simulink library "sixDoFDynamicsCoupled2"  (R2020a)
settings: Solver=VariableStepAuto  StartTime=0.0  StopTime=10.0  RelTol=1e-3
undefined symbols (not defined in the file): vcl
libraries: vrlib x8, eulAng2RotMat_ul x1, eulDot x1
settings Model: Creator=jldanie5  LastModifiedBy=John Jr
settings DataIOCC: ReturnWorkspaceOutputs=off
settings DebuggingCC: ArithmeticOperatorsInVariantConditions=warning
settings SFSimCC: CustomCodeUndefinedFunction=UseInterfaceOnly

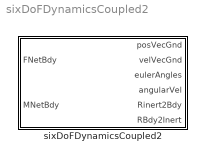
== system sixDoFDynamicsCoupled2 ==
  sixDoFDynamicsCoupled2 : Subsystem  VariantControl=(default)  mask{MMat=vcl.M6x6_B.Value, MaMat=vcl.Ma6x6_LE.Value, rCM_B=vcl.rCM_B.Value, rB_LE=vcl.rB_LE.Value, initPos=vcl.initPosVecGnd.Value, initVel=vcl.initVelVecBdy.Value, initEulAngs=vcl.initEulAng.Value, initAngVel=vcl.initAngVelVec.Value}
      mask prompts: MMat "6x6 Mass Matrix"; MaMat "6x6 Added Mass Matrix"; rCM_B "Center of mass position vec in body frame"; rB_LE "Body frame origin position vec relative to Leading Edge"; initPos "Initial position"; initVel "Initial velocity"; initEulAngs "Initial Euler Angles"; initAngVel "Initial Angular Velocity Vec"
      mask init:
      | S = @(v) [0 -v(3) v(2);v(3) 0 -v(1);-v(2) v(1) 0];
      | MaAdj = [eye(3) zeros(3);-S(rB_LE) eye(3)]*MaMat;
      | MTot = MMat + MaAdj;
      | MTotInv = inv(MTot);
      | 
      | m = MMat(1,1);
      | J = MMat(4:6,4:6);%About Body Frame
      mask DialogControl Container6 Prompt: Mass Matrices
      mask DialogControl Container4 Prompt: Point Locations
      mask DialogControl Container3 Prompt: Initial Conditions

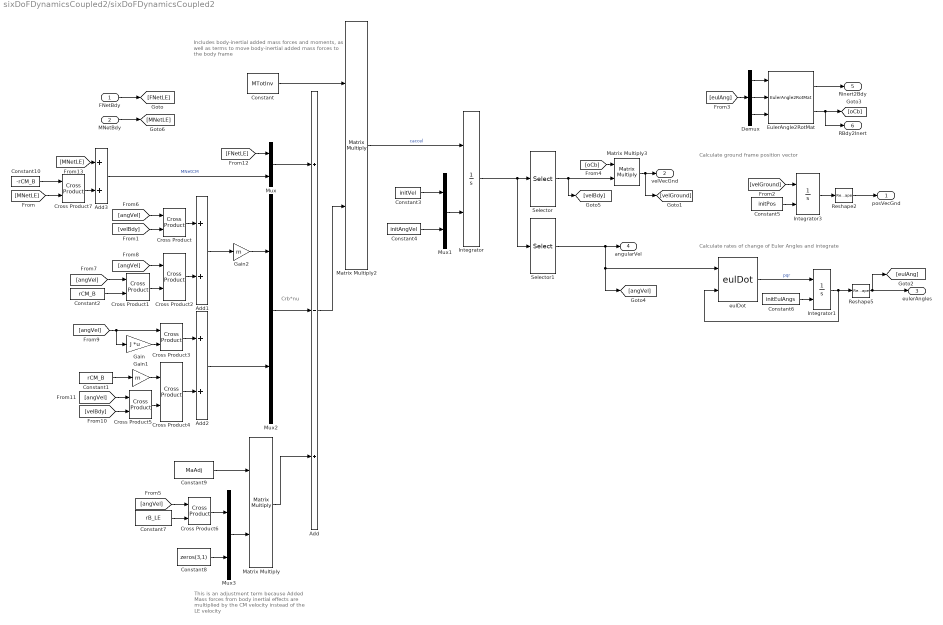
== system sixDoFDynamicsCoupled2/sixDoFDynamicsCoupled2 ==
  note: Crb*nu
  note: This is an adjustment term because Added
      | Mass forces from body inertial effects are
      | multiplied by the CM velocity instead
      | of the LE velocity
  note: Includes body-inertial added mass forces and moments,
      | as well as terms to move body-inertial added mass
      | forces to the body frame
  note: Calculate ground frame position vector
  note: Calculate rates of change of Euler Angles and integrate
  FNetBdy : Inport
  MNetBdy : Inport  Port=2
  Add : Sum  Inputs=+-+
  Add1 : Sum
  Add2 : Sum
  Add3 : Sum
  Constant : Constant  Value=MTotInv  VectorParams1D=off
  Constant1 : Constant  Value=rCM_B
  Constant10 : Constant  Value=-rCM_B  VectorParams1D=off
  Constant2 : Constant  Value=rCM_B
  Constant3 : Constant  Value=initVel
  Constant4 : Constant  Value=initAngVel
  Constant5 : Constant  Value=initPos
  Constant6 : Constant  Value=initEulAngs
  Constant7 : Constant  Value=rB_LE
  Constant8 : Constant  Value=zeros(3,1)
  Constant9 : Constant  Value=MaAdj
  Cross Product{,1..7} (8 alike) : vrlib/Utilities/Cross Product
  Demux : Demux  Outputs=3
  EulerAngle2RotMat : eulAng2RotMat_ul/EulerAngle2RotMat  SystemSampleTime=-1  Latency=0  AutoFrameSizeCalculation=off
  Gain : Gain  Gain=J  Multiplication=Matrix(K*u)
  Gain1 : Gain  Gain=m
  Gain2 : Gain  Gain=m
  Integrator : Integrator  InitialConditionSource=external
  Integrator1 : Integrator  InitialConditionSource=external  InitialCondition=initEulAngs
  Integrator3 : Integrator  InitialConditionSource=external  InitialCondition=initPos
  Matrix Multiply : Product  Multiplication=Matrix(*)
  Matrix Multiply2 : Product  Multiplication=Matrix(*)
  Matrix Multiply3 : Product  Multiplication=Matrix(*)
  Mux{,1..3} (4 alike) : Mux  Inputs=2
  Reshape2 : Reshape  OutputDimensionality=Column vector (2-D)
  Reshape5 : Reshape  OutputDimensionality=Column vector (2-D)
  Selector : Selector  InputPortWidth=6  IndexOptions=Index vector (dialog)  Indices=[1 2 3]  OutputSizes=1
  Selector1 : Selector  InputPortWidth=6  IndexOptions=Index vector (dialog)  Indices=[4 5 6]  OutputSizes=1
  eulDot : eulDot/eulDot  SystemSampleTime=-1  Latency=0  AutoFrameSizeCalculation=off
  posVecGnd : Outport  VectorParamsAs1DForOutWhenUnconnected=off
  velVecGnd : Outport  Port=2  VectorParamsAs1DForOutWhenUnconnected=off
  eulerAngles : Outport  Port=3  VectorParamsAs1DForOutWhenUnconnected=off
  angularVel : Outport  Port=4  VectorParamsAs1DForOutWhenUnconnected=off
  Rinert2Bdy : Outport  Port=5  VectorParamsAs1DForOutWhenUnconnected=off
  RBdy2Inert : Outport  Port=6  VectorParamsAs1DForOutWhenUnconnected=off
  wires:
  Mux/1 -> Add/1
  Constant/1 -> Matrix Multiply2/1
  Matrix Multiply2/1 -> Integrator/1  "caccel"
  Integrator/1 -> Selector1/1, Selector/1
  Constant4/1 -> Mux1/2
  Mux1/1 -> Integrator/2
  Integrator3/1 -> Reshape2/1
  Demux/3 -> EulerAngle2RotMat/3
  Demux/1 -> EulerAngle2RotMat/1
  EulerAngle2RotMat/2 -> RBdy2Inert/1, [oCb]
  Reshape2/1 -> posVecGnd/1
  Demux/2 -> EulerAngle2RotMat/2
  Constant5/1 -> Integrator3/2
  [eulAng] -> Demux/1
  eulDot/1 -> Integrator1/1  "pqr"
  Integrator1/1 -> Reshape5/1, eulDot/2
  Constant6/1 -> Integrator1/2
  Reshape5/1 -> eulerAngles/1, [eulAng]
  Selector1/1 -> [angVel], eulDot/1, angularVel/1
  [velGround] -> Integrator3/1
  EulerAngle2RotMat/1 -> Rinert2Bdy/1
  Constant3/1 -> Mux1/1
  Selector/1 -> [velBdy], Matrix Multiply3/2
  [oCb] -> Matrix Multiply3/1
  Matrix Multiply3/1 -> [velGround], velVecGnd/1
  Mux2/1 -> Add/2
  [velBdy] -> Cross Product/2
  [angVel] -> Cross Product/1
  Cross Product/1 -> Add1/1
  Cross Product1/1 -> Cross Product2/2
  Constant2/1 -> Cross Product1/2
  [angVel] -> Cross Product1/1
  [angVel] -> Cross Product2/1
  Cross Product2/1 -> Add1/2
  [angVel] -> Cross Product3/1, Gain/1
  Gain/1 -> Cross Product3/2
  Constant1/1 -> Gain1/1
  Gain1/1 -> Cross Product4/1
  [velBdy] -> Cross Product5/2
  [angVel] -> Cross Product5/1
  Cross Product5/1 -> Cross Product4/2
  Cross Product3/1 -> Add2/1
  Cross Product4/1 -> Add2/2
  Add1/1 -> Gain2/1
  Add2/1 -> Mux2/2
  Add/1 -> Matrix Multiply2/2
  Gain2/1 -> Mux2/1
  Matrix Multiply/1 -> Add/3
  [angVel] -> Cross Product6/1
  Constant7/1 -> Cross Product6/2
  Cross Product6/1 -> Mux3/1
  Constant8/1 -> Mux3/2
  Mux3/1 -> Matrix Multiply/2
  Constant9/1 -> Matrix Multiply/1
  FNetBdy/1 -> [FNetLE]
  MNetBdy/1 -> [MNetLE]
  [FNetLE] -> Mux/1
  [MNetLE] -> Cross Product7/2
  Constant10/1 -> Cross Product7/1
  [MNetLE] -> Add3/1
  Cross Product7/1 -> Add3/2
  Add3/1 -> Mux/2  "MNetCM"
